simulink model "bh_ssc_mech_BEGIN"  (R2018a)
settings: Solver=VariableStepAuto  StartTime=0.0  StopTime=3  MaxStep=0.01  RelTol=1e-3  AbsTol=1e-3  EnableMultiTasking=on
libraries: nesl_utility x6, fl_lib x4
CloseFcn:
  | try,close(h1_ssc_solenoid),end
  | clear h1_ssc_solenoid
  | 
  | clear simlog_ssc_solenoid
Description:
  | Solenoid
  | 
  | Copyright 2008-2017 The MathWorks, Inc.
settings Model: Creator=MathWorks  LastModifiedBy=bhorton
settings SolverCC: AutoScaleAbsTol=off
settings DataIOCC: LimitDataPoints=on  SaveFormat=Array
settings OptimizationCC: LifeSpan=inf
settings DebuggingCC: SolverPrmCheckMsg=warning  AllowSymbolicDim=off  SFUnexpectedBacktrackingDiag=warning  SFNoUnconditionalDefaultTransitionDiag=warning  SFExecutionAtInitializationDiag=none
settings HardwareCC: ProdBitPerPointer=32  ProdBitPerSizeT=32  ProdBitPerPtrDiffT=32  ProdLargestAtomicFloat=None  ProdIntDivRoundTo=Undefined  ProdEndianess=Unspecified  ProdWordSize=32  ProdHWDeviceType=32-bit Generic
settings ModelReferenceCC: PropagateSignalLabelsOutOfModel=off
settings CodeAppCC: StateflowObjectComments=on
settings GRTTargetCC: TargetLangStandard=C89/C90 (ANSI)  GeneratePreprocessorConditionals=Disable all
settings ConfigComp: CovMetricSettings=dw  CovHtmlReporting=on  CovSaveCumulativeToWorkspaceVar=on  CovSaveSingleToWorkspaceVar=on  CovExternalEMLEnable=off  CovSFcnEnable=off
settings SimscapeCC: SimscapeLogType=all  SimscapeLogSimulationStatistics=on  SimscapeLogName=simlog_ssc_solenoid  SimscapeLogDataHistory=10000

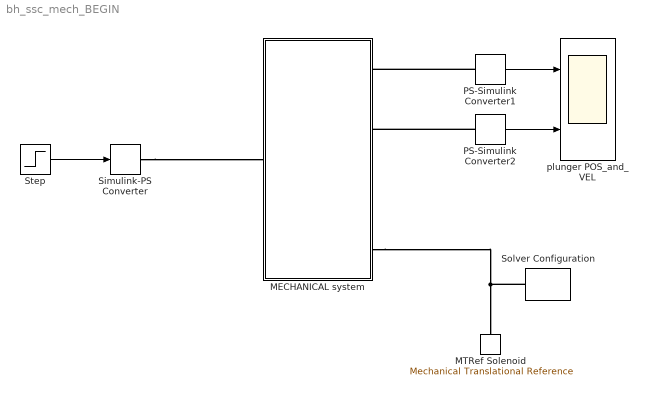
== system bh_ssc_mech_BEGIN ==
  MECHANICAL system : Subsystem
  MTRef Solenoid : fl_lib/Mechanical/Translational Elements/Mechanical Translational Reference
  PS-Simulink Converter1 : nesl_utility/PS-Simulink Converter  PhysicalDomain=network_engine_domain  SubClassName=ps_output  LeftPortType=input  RightPortType=output  PseudoPeriodic=off  Frequencies=[]  Unit=m  AffineConversion=off
      settings: AttributesFormatString=units=%<Unit>
  PS-Simulink Converter2 : nesl_utility/PS-Simulink Converter  PhysicalDomain=network_engine_domain  SubClassName=ps_output  LeftPortType=input  RightPortType=output  PseudoPeriodic=off  Frequencies=[]  Unit=m/s  AffineConversion=off
      settings: AttributesFormatString=units=%<Unit>
  Simulink-PS Converter : nesl_utility/Simulink-PS Converter  PhysicalDomain=network_engine_domain  SubClassName=ps_input  LeftPortType=input  RightPortType=output  PseudoPeriodic=off  Frequencies=[]  NoiseDistribution=none  NoiseParameters=[]  Unit=N  AffineConversion=off  FilteringAndDerivatives=provide  SimscapeFilterOrder=1  InputFilterTimeConstant=0.001  UdotUserProvided=0
  Solver Configuration : nesl_utility/Solver Configuration  PhysicalDomain=network_engine_domain  SubClassName=solver  LeftPortType=input  RightPortType=generic  Tones=[]  Harmonics=[]  SimulateNoise=off  Profile=off  UseLocalSampling=off  EnableSwitchedLinearOptims=on  FrequencyDomain=off  UseCCode=off  RelTol=0.001  AbsTol=1e-06  MinStep=1e-09  ToWorkspace=off  RevertToSquareIcSolve=off  NumHomotopyIterations=100  PhasorMode=off  PhasorModeNumHarmonics=1  DoDC=off  ResidualTolerance=1e-09  UseLocalSolver=off  LocalSolverChoice=NE_BACKWARD_EULER_ADVANCER  LocalSolverSampleTime=0.001  DoFixedCost=off  MaxNonlinIter=3  MaxModeIter=2  LinearAlgebra=Sparse  EquationFormulation=NE_TIME_EF  DelaysMemoryBudget=1024  AutomaticFiltering=on  FilteringTimeConstant=0.001
  Step : Step  SampleTime=0
  plunger POS_and_VEL : Scope  NumInputPorts=2
  wires:
  PS-Simulink Converter1/1 -> plunger POS_and_VEL/1
  PS-Simulink Converter2/1 -> plunger POS_and_VEL/2
  Step/1 -> Simulink-PS Converter/1
  connections:
  PS-Simulink Converter1/LConn1 -- MECHANICAL system/RConn1
  PS-Simulink Converter2/LConn1 -- MECHANICAL system/RConn2
  MECHANICAL system/RConn4 -- Solver Configuration/RConn1 -- MTRef Solenoid/LConn1
  Simulink-PS Converter/RConn1 -- MECHANICAL system/LConn1

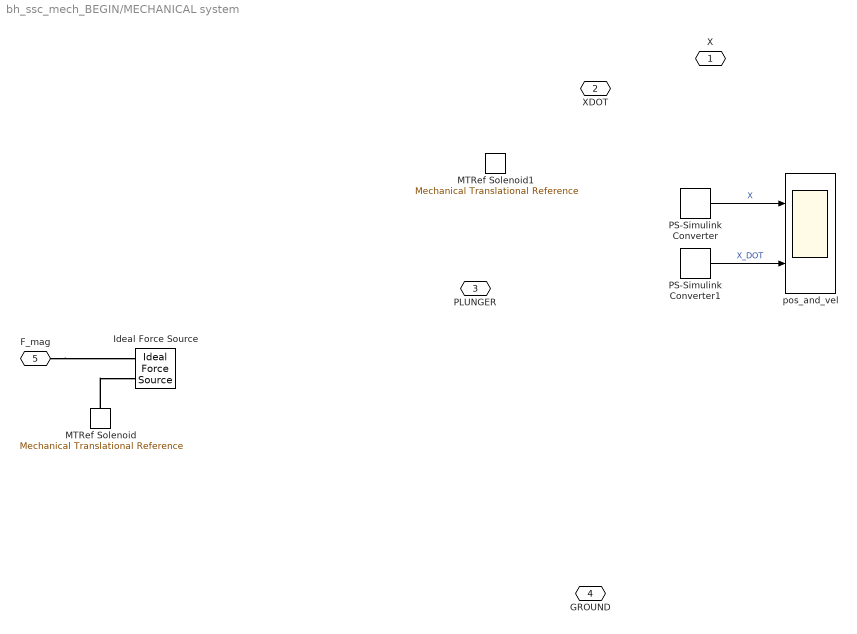
== system bh_ssc_mech_BEGIN/MECHANICAL system ==
  Ideal Force Source : fl_lib/Mechanical/Mechanical Sources/Ideal Force Source
  MTRef Solenoid : fl_lib/Mechanical/Translational Elements/Mechanical Translational Reference
  MTRef Solenoid1 : fl_lib/Mechanical/Translational Elements/Mechanical Translational Reference
  PS-Simulink Converter : nesl_utility/PS-Simulink Converter  PhysicalDomain=network_engine_domain  SubClassName=ps_output  LeftPortType=input  RightPortType=output  PseudoPeriodic=off  Frequencies=[]  Unit=m  AffineConversion=off
      settings: AttributesFormatString=unit=%<Unit>
  PS-Simulink Converter1 : nesl_utility/PS-Simulink Converter  PhysicalDomain=network_engine_domain  SubClassName=ps_output  LeftPortType=input  RightPortType=output  PseudoPeriodic=off  Frequencies=[]  Unit=m/s  AffineConversion=off
      settings: AttributesFormatString=unit=%<Unit>
  pos_and_vel : Scope  NumInputPorts=2
  X : PMIOPort  Side=Right
  XDOT : PMIOPort  Port=2  Side=Right
  PLUNGER : PMIOPort  Port=3  Side=Right
  GROUND : PMIOPort  Port=4  Side=Right
  F_mag : PMIOPort  Port=5  Side=Left
  wires:
  PS-Simulink Converter/1 -> pos_and_vel/1  "X"
  PS-Simulink Converter1/1 -> pos_and_vel/2  "X_DOT"
  connections:
  F_mag/RConn1 -- Ideal Force Source/RConn1
  MTRef Solenoid/LConn1 -- Ideal Force Source/RConn2
